simulink model "FixedWingLowFidelity"  (R2024a)
settings: Solver=VariableStepAuto  StartTime=0.0  StopTime=10.0  RelTol=1e-3
undefined symbols (not defined in the file): AirSpeed, Gravity, Height, RollAngle, WindDown, WindEast, WindNorth
libraries: uavalgslib x1
settings Model: Creator=hrish  LastModifiedBy=hrish

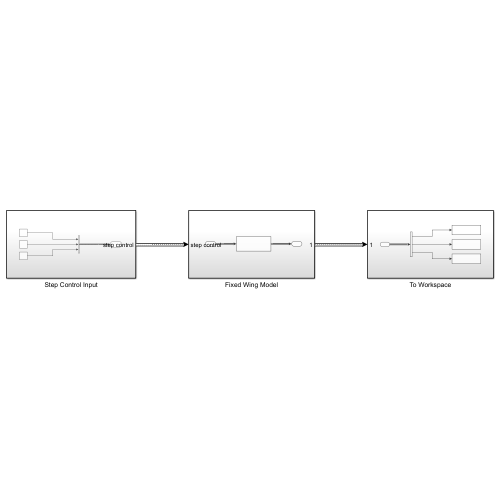
[thumbnail: Simulink's stored preview of the top-level diagram]
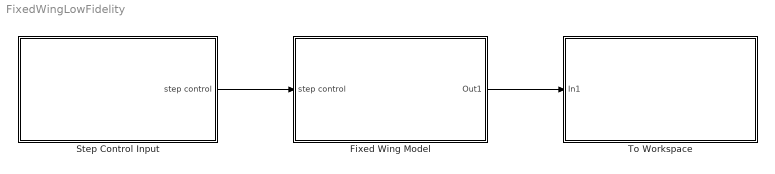
== system FixedWingLowFidelity ==
  Fixed Wing Model : Subsystem
  Step Control Input : Subsystem
  To Workspace : Subsystem
  wires:
  Step Control Input/1(step control) -> Fixed Wing Model/1(step control)
  Fixed Wing Model/1(Out1) -> To Workspace/1(In1)

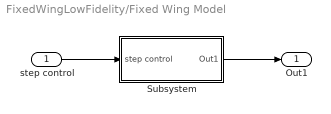
== system FixedWingLowFidelity/Fixed Wing Model ==
  step control : Inport
  Subsystem : Subsystem
  Out1 : Outport
  wires:
  step control/1 -> Subsystem/1(step control)
  Subsystem/1(Out1) -> Out1/1

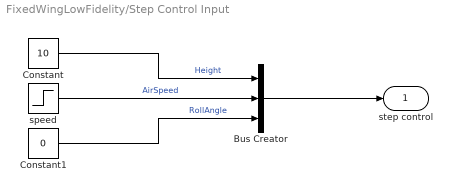
== system FixedWingLowFidelity/Step Control Input ==
  Bus Creator : BusCreator  Inputs=Height,AirSpeed,RollAngle  OutDataTypeStr=Bus: FixedWingGuidanceControlBus  NonVirtualBus=on
  Constant : Constant  Value=10
  Constant1 : Constant  Value=0
  speed : Step  SampleTime=0
  step control : Outport
  wires:
  speed/1 -> Bus Creator/2  "AirSpeed"
  Constant/1 -> Bus Creator/1  "Height"
  Constant1/1 -> Bus Creator/3  "RollAngle"
  Bus Creator/1 -> step control/1

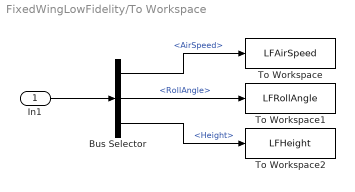
== system FixedWingLowFidelity/To Workspace ==
  In1 : Inport
  Bus Selector : BusSelector  OutputSignals=AirSpeed,RollAngle,Height
  To Workspace : ToWorkspace  VariableName=LFAirSpeed  SaveFormat=Timeseries  SampleTime=-1
  To Workspace1 : ToWorkspace  VariableName=LFRollAngle  SaveFormat=Timeseries  SampleTime=-1
  To Workspace2 : ToWorkspace  VariableName=LFHeight  SaveFormat=Timeseries  SampleTime=-1
  wires:
  In1/1 -> Bus Selector/1
  Bus Selector/1 -> To Workspace/1  "<AirSpeed>"
  Bus Selector/2 -> To Workspace1/1  "<RollAngle>"
  Bus Selector/3 -> To Workspace2/1  "<Height>"

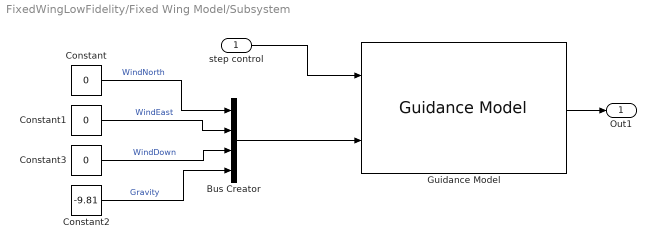
== system FixedWingLowFidelity/Fixed Wing Model/Subsystem ==
  step control : Inport
  Bus Creator : BusCreator  Inputs=WindNorth,WindEast,WindDown,Gravity  OutDataTypeStr=Bus: FixedWingGuidanceEnvironmentBus  NonVirtualBus=on
  Constant : Constant  Value=0
  Constant1 : Constant  Value=0
  Constant2 : Constant  Value=-9.81
  Constant3 : Constant  Value=0
  Guidance Model : uavalgslib/Guidance Model  ModelType=FixedWingGuidance  SpecifiedDataType=double  SimulateUsing=Interpreted execution  InitialWorldPositionMultirotor=[0; 0; 0]  InitialWorldVelocityMultirotor=[0; 0; 0]  InitialEulerZYXMultirotor=[0; 0; 0]  InitialBodyAngularRateRPYMultirotor=[0; 0; 0]  InitialThrustMultirotor=0  InitialNorthFixedWing=0  InitialEastFixedWing=0  InitialHeightFixedWing=0  InitialAirSpeedFixedWing=0  InitialHeadingAngleFixedWing=0  InitialFlightPathAngleFixedWing=0  InitialRollAngleFixedWing=0  InitialRollAngleRateFixedWing=0  PDRollMultirotor=[3402.97,116.67]  PDPitchMultirotor=[3402.97, 116.67]  PYawRateMultirotor=1950  PThrustMultirotor=3900  MassMultirotor=0.1  PHeightFixedWing=3.9  PHeadingAngleFixedWing=3.9  PFlightPathAngleFixedWing=39  PDRollFixedWing=[3402.97, 116.67]  PAirSpeedFixedWing=1  FlightPathAngleLimitsFixedWing=[-pi/2, pi/2]  StateBusName='FixedWingGuidanceStateBus'  ControlBusName='FixedWingGuidanceControlBus'  EnvironmentBusName='FixedWingGuidanceEnvironmentBus'  DataType=double
  Out1 : Outport
  wires:
  Constant/1 -> Bus Creator/1  "WindNorth"
  Constant1/1 -> Bus Creator/2  "WindEast"
  Constant3/1 -> Bus Creator/3  "WindDown"
  Constant2/1 -> Bus Creator/4  "Gravity"
  step control/1 -> Guidance Model/1
  Bus Creator/1 -> Guidance Model/2
  Guidance Model/1 -> Out1/1
